simulink model "functionTest"  (R2021a)
settings: Solver=FixedStepAuto  StartTime=0.0  StopTime=30  RelTol=1e-3
settings Model: Creator=seedship  LastModifiedBy=seedship
settings SolverCC: AlgebraicLoopSolver=TrustRegion
settings DebuggingCC: SFMachineParentedDataDiag=warning

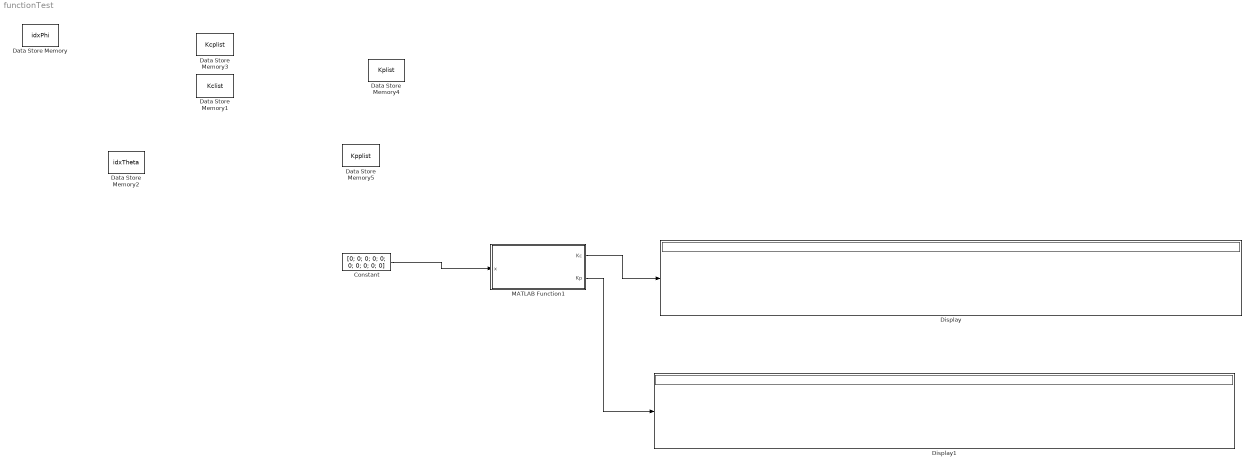
== system functionTest ==
  Constant : Constant  Value=[0; 0; 0; 0; 0; 0; 0; 0; 0; 0]
  Data Store Memory : DataStoreMemory  DataStoreName=idxPhi  ReadBeforeWriteMsg=warning  WriteAfterWriteMsg=warning  WriteAfterReadMsg=warning  InitialValue=idxPhi  VectorParams1D=off  ShowAdditionalParam=off  OutDataTypeStr=double
  Data Store Memory1 : DataStoreMemory  DataStoreName=Kclist  ReadBeforeWriteMsg=warning  WriteAfterWriteMsg=warning  WriteAfterReadMsg=warning  InitialValue=Kclist  VectorParams1D=off  ShowAdditionalParam=off  OutDataTypeStr=double
  Data Store Memory2 : DataStoreMemory  DataStoreName=idxTheta  ReadBeforeWriteMsg=warning  WriteAfterWriteMsg=warning  WriteAfterReadMsg=warning  InitialValue=idxTheta  ShowAdditionalParam=off  OutDataTypeStr=double
  Data Store Memory3 : DataStoreMemory  DataStoreName=Kcplist  ReadBeforeWriteMsg=warning  WriteAfterWriteMsg=warning  WriteAfterReadMsg=warning  InitialValue=Kcplist  ShowAdditionalParam=off  OutDataTypeStr=double
  Data Store Memory4 : DataStoreMemory  DataStoreName=Kplist  ReadBeforeWriteMsg=warning  WriteAfterWriteMsg=warning  WriteAfterReadMsg=warning  InitialValue=Kplist  ShowAdditionalParam=off  OutDataTypeStr=double
  Data Store Memory5 : DataStoreMemory  DataStoreName=Kpplist  ReadBeforeWriteMsg=warning  WriteAfterWriteMsg=warning  WriteAfterReadMsg=warning  InitialValue=Kpplist  ShowAdditionalParam=off  OutDataTypeStr=double
  Display : Display
  Display1 : Display
  MATLAB Function1 : MATLAB Function  TreatAsAtomicUnit=on
  wires:
  MATLAB Function1/1(Kc) -> Display/1
  Constant/1 -> MATLAB Function1/1(x)
  MATLAB Function1/2(Kp) -> Display1/1

== matlab function functionTest/MATLAB Function1 ==
  data: x input; Kc output size=[4 12]; Kp output size=[2 16]; idxPhi data_store_memory; Kclist data_store_memory; Kplist data_store_memory; idxTheta data_store_memory; Kcplist data_store_memory; Kpplist data_store_memory
function [Kc, Kp] = calculateRSLQRGains(x)
    % Nearest A, B
    global idxPhi idxTheta Kclist Kplist Kcplist Kpplist
    [~, idx] = min(abs(x(8) - idxPhi));
    
    selectSizeC = 4;
    selectSizeP = 2;
    
    if idx ~= ceil(length(idxPhi)/2)
        Kc = Kclist(selectSizeC*(idx-1)+1:selectSizeC*idx,:);
        Kp = Kplist(selectSizeP*(idx-1)+1:selectSizeP*idx,:);
        return
    end
    
    [~, idx] = min(abs(x(4) - idxTheta));
    Kc = Kcplist(selectSizeC*(idx-1)+1:selectSizeC*idx,:);
    Kp = Kpplist(selectSizeP*(idx-1)+1:selectSizeP*idx,:);
end
